simulink model "basic_sliding_mode"  (R2020a)
settings: Solver=VariableStepAuto  StartTime=0.0  StopTime=10.0  RelTol=1e-3
settings Model: Creator=ripme  LastModifiedBy=ripme
settings SolverCC: ZeroCrossAlgorithm=Adaptive
settings DebuggingCC: IgnoredZcDiagnostic=none

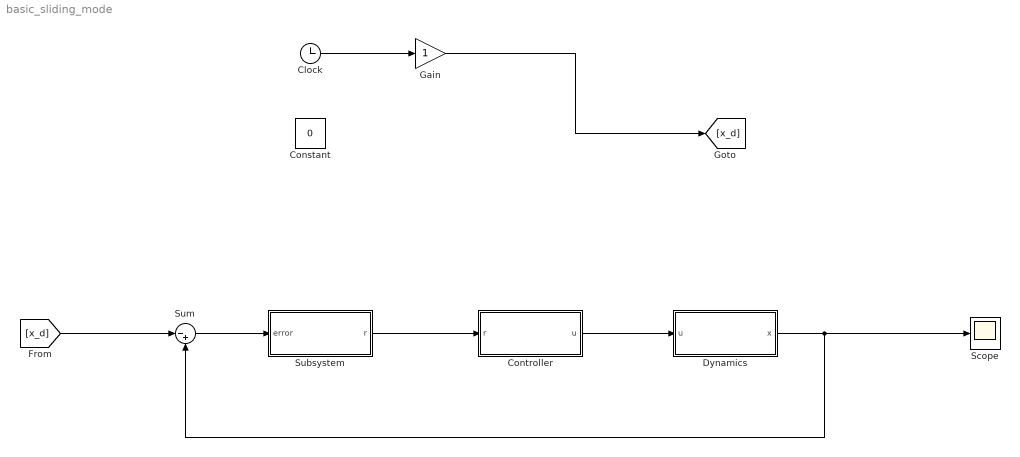
== system basic_sliding_mode ==
  Clock : Clock
  Constant : Constant  Value=0
  Controller : Subsystem
  Dynamics : Subsystem
  Gain : Gain
  Scope : Scope
  Subsystem : Subsystem
  Sum : Sum  Inputs=|-+
  wires:
  Controller/1(u) -> Dynamics/1(u)
  [x_d] -> Sum/1
  Dynamics/1(x) -> Scope/1, Sum/2
  Gain/1 -> [x_d]
  Clock/1 -> Gain/1
  Subsystem/1(r) -> Controller/1(r)
  Sum/1 -> Subsystem/1(error)

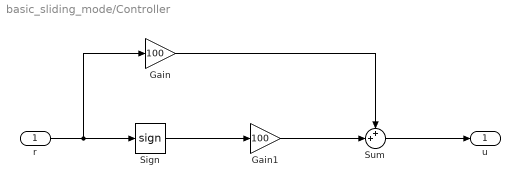
== system basic_sliding_mode/Controller ==
  r : Inport
  Gain : Gain  Gain=100
  Gain1 : Gain  Gain=100
  Sign : Signum
  Sum : Sum  Inputs=++|
  u : Outport
  wires:
  Sum/1 -> u/1
  Gain/1 -> Sum/1
  Gain1/1 -> Sum/2
  Sign/1 -> Gain1/1
  r/1 -> Gain/1, Sign/1

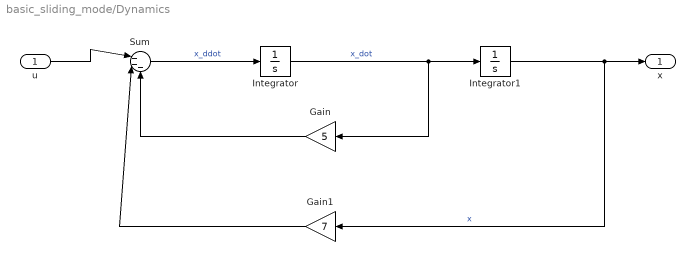
== system basic_sliding_mode/Dynamics ==
  u : Inport
  Gain : Gain  Gain=5
  Gain1 : Gain  Gain=7
  Integrator : Integrator  InitialCondition=20
  Integrator1 : Integrator  InitialCondition=20
  Sum : Sum  Inputs=|---
  x : Outport
  wires:
  Sum/1 -> Integrator/1  "x_ddot"
  Integrator/1 -> Gain/1, Integrator1/1  "x_dot"
  Integrator1/1 -> Gain1/1, x/1  "x"
  u/1 -> Sum/1
  Gain/1 -> Sum/3
  Gain1/1 -> Sum/2

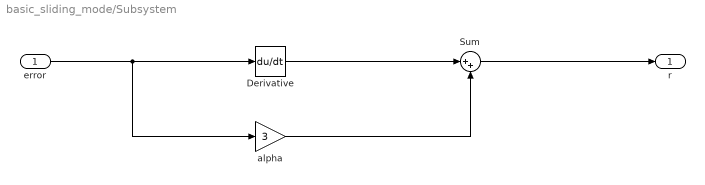
== system basic_sliding_mode/Subsystem ==
  error : Inport
  Derivative : Derivative
  Sum : Sum  Inputs=|++
  alpha : Gain  Gain=3
  r : Outport
  wires:
  alpha/1 -> Sum/2
  Sum/1 -> r/1
  Derivative/1 -> Sum/1
  error/1 -> alpha/1, Derivative/1
